simulink model "untitled"  (R2016a)
settings: Solver=VariableStepAuto  StartTime=0.0  StopTime=10.0  RelTol=1e-3
settings Model: Creator=kreitzem  LastModifiedBy=kreitzem

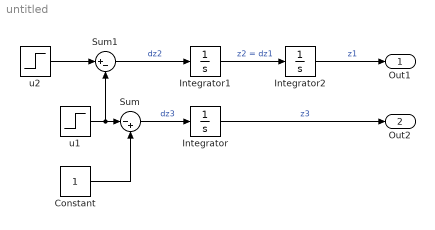
== system untitled ==
  Constant : Constant
  Integrator : Integrator
  Integrator1 : Integrator
  Integrator2 : Integrator
  Sum : Sum  Inputs=|-+
  Sum1 : Sum  Inputs=|+-
  u1 : Step  SampleTime=0
  u2 : Step  SampleTime=0
  Out1 : Outport
  Out2 : Outport  Port=2
  wires:
  u1/1 -> Sum1/2, Sum/1
  Constant/1 -> Sum/2
  Sum/1 -> Integrator/1  "dz3"
  u2/1 -> Sum1/1
  Sum1/1 -> Integrator1/1  "dz2"
  Integrator1/1 -> Integrator2/1  "z2 = dz1"
  Integrator/1 -> Out2/1  "z3"
  Integrator2/1 -> Out1/1  "z1"
